simulink model "ProvaXsens"  (R2017b)
settings: Solver=FixedStepAuto  StartTime=0.0  StopTime=Inf  RelTol=1e-3
libraries: XsensLibrary x3, robotcorelib x1
settings Model: SimulationMode=external  ExtModeTrigDuration=10000  Creator=constantin  LastModifiedBy=root
settings DataIOCC: LimitDataPoints=on  SaveFormat=Array
settings OptimizationCC: ExpressionDepthLimit=2147483647  LifeSpan=1
settings DebuggingCC: UnderspecifiedInitializationDetection=Classic  MergeDetectMultiDrivingBlocksExec=none  SolverPrmCheckMsg=warning  StateNameClashWarn=warning  SFUnexpectedBacktrackingDiag=warning  SFNoUnconditionalDefaultTransitionDiag=warning  SFExecutionAtInitializationDiag=none
settings HardwareCC: ProdBitPerPointer=32  ProdBitPerSizeT=32  ProdBitPerPtrDiffT=32  ProdLargestAtomicFloat=None  ProdIntDivRoundTo=Undefined  ProdEndianess=Unspecified  ProdWordSize=32  ProdHWDeviceType=32-bit Generic
settings ModelReferenceCC: PropagateSignalLabelsOutOfModel=off
settings SFSimCC: SimCustomHeaderCode="#include \"rehamove.hpp\""  MATLABDynamicMemAlloc=off
settings SFSimCC: SimUserIncludeDirs=|
  | /Users/constantin/Documents/retrainer/retrainer.repo/code/trunk/incl/rehamove/
  | /Users/constantin/Documents/retrainer/retrainer.repo/code/trunk/incl/
settings RTWCC: SystemTargetFile=ert_linux.tlc  MakeCommand=make_rtw OPTS=-DWITH_HW OPTIMIZATION_FLAGS=-O3  TemplateMakefile=ert_linux.tmf  Description=Linux Embedded Coder  TargetLang=C++
settings CodeAppCC: IgnoreCustomStorageClasses=off  CustomSymbolStrType=$N$R$M  StateflowObjectComments=on  InternalIdentifier=Classic
settings STFCustomTargetCC: ModelReferenceCompliant=off  CombineOutputUpdateFcns=on  ERTCustomFileBanners=on  SupportComplex=off  RemoveResetFunc=on  SupportVariableSizeSignals=on  MATLABClassNameForMDSCustomization=Simulink.SoftwareTarget.ERTCustomization  GRTInterface=off  SystemTargetFile=ert_linux.tlc
settings ERTTargetCC: MultiwordLength=2048  ModelReferenceCompliant=off  ParMdlRefBuildCompliant=off  CompOptLevelCompliant=off  ConcurrentExecutionCompliant=off  SupportComplex=off  SupportContinuousTime=on  SupportNonInlinedSFcns=on  SupportVariableSizeSignals=on  ModelStepFunctionPrototypeControlCompliant=off  CPPClassGenCompliant=off  UseToolchainInfoCompliant=off  ExtMode=on  MultiInstanceErrorCode=None  ERTCustomFileTemplate=ert_linux_file_process.tlc  ConvertIfToSwitch=off  SuppressUnreachableDefaultCases=off
settings ConfigComp: CovMetricSettings=dw  CovHtmlReporting=on  CovSaveCumulativeToWorkspaceVar=on  CovSaveSingleToWorkspaceVar=on  CovExternalEMLEnable=off  CovSFcnEnable=off
settings SimscapeCC: SimscapeNormalizeSystem=off
settings ConfigurationSet: Description=SimMechanics 2G

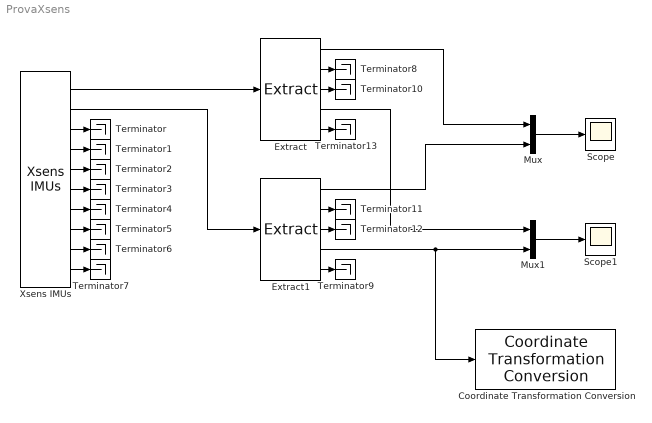
== system ProvaXsens ==
  Coordinate Transformation Conversion : robotcorelib/Coordinate Transformation Conversion  InputRepresentation=Quaternion  InputEulerSequence=ZYX  ShowTrVecInputPort=on  OutputRepresentation=Rotation Matrix  OutputEulerSequence=ZYX  ShowTrVecOutputPort=on  SimulateUsing=Code generation
      settings: SourceProductBaseCode=RO
  Extract : XsensLibrary/Extract  correction=off
  Extract1 : XsensLibrary/Extract  correction=off
  Mux : Mux  Inputs=2
  Mux1 : Mux  Inputs=2
  Scope : Scope
  Scope1 : Scope
  Terminator{,1..13} (14 alike) : Terminator
  Xsens IMUs : XsensLibrary/Xsens IMUs  SID00='/dev/Xsens'  SID01='00B419BB'  SID02='00B419B5'  SID03='0'  SID04='0'  SID05='0'  SID06='0'  SID07='0'  SID08='0'  SID09='0'  SID10='0'  Freq=120  Ts=0.01  UseCalibratedValues=on
  wires:
  Xsens IMUs/1 -> Extract/1
  Extract/1 -> Mux/1
  Extract/4 -> Mux1/1
  Extract1/1 -> Mux/2
  Extract1/4 -> Coordinate Transformation Conversion/1, Mux1/2
  Xsens IMUs/2 -> Extract1/1
  Xsens IMUs/3 -> Terminator/1
  Xsens IMUs/4 -> Terminator1/1
  Xsens IMUs/5 -> Terminator2/1
  Xsens IMUs/6 -> Terminator3/1
  Xsens IMUs/7 -> Terminator4/1
  Xsens IMUs/8 -> Terminator5/1
  Xsens IMUs/9 -> Terminator6/1
  Xsens IMUs/10 -> Terminator7/1
  Extract/2 -> Terminator8/1
  Extract/3 -> Terminator10/1
  Extract1/2 -> Terminator11/1
  Extract1/3 -> Terminator12/1
  Mux/1 -> Scope/1
  Mux1/1 -> Scope1/1
  Extract1/5 -> Terminator9/1
  Extract/5 -> Terminator13/1
